simulink model "full_maneuver_platoon"  (R2022a)
settings: Solver=ode23t  StartTime=0.0  StopTime=300  FixedStep=0.1  MaxStep=0.01  RelTol=1e-3
InitFcn:
  | totalVehicles = 7;
  | if exist('vehStatesBus', 'var')==0
  | load vehBuses
  | end
  | if exist('vehErrorsBus', 'var')==0
  | load vehBuses
  | end
libraries: simulink x80, powerlib_meascontrol x16, autolibshared x7, dspsigops x4
(part 2 of 9)

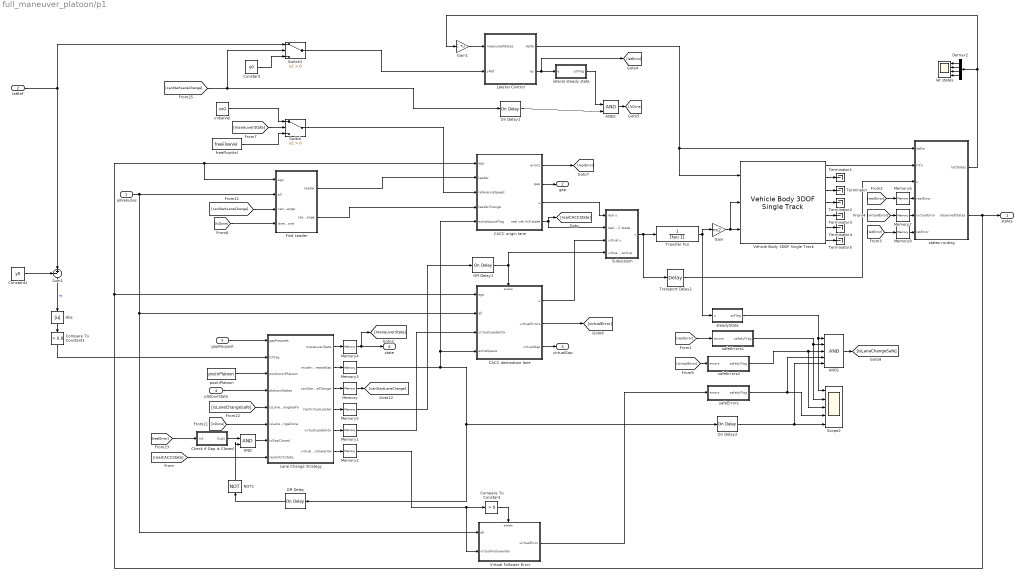
== system full_maneuver_platoon/p1 ==
  allVehicles : Inport
  latRef : Inport  Port=2
  gapRequest : Inport  Port=3
  platoonState : Inport  Port=4
  AND : Logic  IconShape=distinctive  AllPortsSameDT=off  OutDataTypeStr=boolean
  AND1 : Logic  Inputs=5  IconShape=distinctive  AllPortsSameDT=off  OutDataTypeStr=boolean
  AND2 : Logic  IconShape=distinctive  AllPortsSameDT=off  OutDataTypeStr=boolean
  Abs : Abs  SaturateOnIntegerOverflow=off
  CACC destination lane : Subsystem
  CACC origin lane : Subsystem
  Check if Gap is Closed : Subsystem
  Compare To Constant : simulink/Logic and Bit Operations/Compare To Constant  relop=>  const=0  OutDataTypeStr=boolean
  Compare To Constant1 : simulink/Logic and Bit Operations/Compare To Constant  relop=>  const=0.8  OutDataTypeStr=boolean
  Constant : Constant  Value=y0
  Constant1 : Constant  Value=y0
  Demux2 : Demux
  Find Leader : Subsystem
  Gain : Gain  Gain=m/2
  Gain1 : Gain  Gain=C  Multiplication=Matrix(K*u)
  Lane Change Strategy : Subsystem  Variant=on  VariantControlMode=label  LabelModeActiveChoice=leaderFirstInvert
  Lateral Control : Subsystem
  Memory{,1..8} (9 alike) : Memory
  NOT1 : Logic  Operator=NOT  IconShape=distinctive  AllPortsSameDT=off  OutDataTypeStr=boolean
  Off Delay : powerlib_meascontrol/Logic/On Delay  DelayType=Off delay  delay=1  ic=0  Ts=0
  Off Delay1 : powerlib_meascontrol/Logic/On Delay  DelayType=Off delay  delay=1  ic=0  Ts=0
  On Delay1 : powerlib_meascontrol/Logic/On Delay  DelayType=On delay  delay=1  ic=0  Ts=0
  On Delay2 : powerlib_meascontrol/Logic/On Delay  DelayType=On delay  delay=1  ic=0  Ts=0
  Scope2 : Scope  NumInputPorts=5
  Subsystem : Subsystem
  Sum1 : Sum  Inputs=-+|
  Switch : Switch  Criteria=u2 > Threshold  SaturateOnIntegerOverflow=off  InputSameDT=off
  Switch1 : Switch  Criteria=u2 > Threshold  SaturateOnIntegerOverflow=off  InputSameDT=off
  Terminator{,1..5} (6 alike) : Terminator
  Transfer Fcn : TransferFcn  Denominator=[tau 1]
  Transport Delay1 : TransportDelay  DelayTime=0.01
  Vehicle Body 3DOF Single Track : autolibshared/Vehicle Body 3DOF Single Track  trackMode=Single (bicycle)  inputMode=External longitudinal forces  frontSteerMode=on  rearSteerMode=off  windMode=off  muMode=off  extFMode=off  extMMode=off  htchFMode=off  htchMMode=off  extXo=off  extpsio=off  extxdoto=off  extro=off  extYo=off  extTamb=off  extydoto=off  aMode=2  NF=2  NR=2  m=m  a=lf  b=lr  h=0.35  dh=1  hh=0.2  X_o=x0  xdot_o=vx0  CalphaMode=off  sigmaMode=on  d=0  hl=0  w=[1.4,1.4]  Cy_f=12e3  Cy_r=11e3  sigma_f=.1  sigma_r=.1  alpha_f_brk=[-.1 .1]  Cy_f_data=[-9e3 9e3]  alpha_r_brk=[-.1 .1]  Cy_r_data=[-9e3 9e3]  Y_o=y0  ydot_o=0  Izz=4000  psi_o=0  r_o=0  Af=2  Cd=.3  Cl=.1  Cpm=.1  beta_w=[0:0.01:0.3]  Cs=[0:0.03:0.9]  Cym=[0:0.01:0.3]  Pabs=101325  Tair=273  g=9.81  mu=1  xdot_tol=.01  Fznom=5000  Fxtire_sat=7e4  Fytire_sat=7e4  longOff=0  latOff=0  vertOff=0  wrapAng=off
      settings: SourceProductBaseCode=PW,DR,MT,VE
  Virtual Follower Error : Subsystem  TreatAsAtomicUnit=on
  freeFlowVel : Constant  Value=freeFlowVel
  initialVel : Constant  Value=vx0
  lat states : Scope  NumInputPorts=4
  lateral steady state : Subsystem
  posInPlatoon : Constant  Value=posInPlatoon
  safeErrors : Subsystem
  safeErrors1 : Subsystem
  safeErrors2 : Subsystem
  states routing : Subsystem
  steadyState : Subsystem
  states : Outport  VectorParamsAs1DForOutWhenUnconnected=off
  gap : Outport  Port=2  VectorParamsAs1DForOutWhenUnconnected=off
  virtualGap : Outport  Port=3  VectorParamsAs1DForOutWhenUnconnected=off
  state : Outport  Port=4  VectorParamsAs1DForOutWhenUnconnected=off
  wires:
  [realCACCState] -> Lane Change Strategy/8(realCACCstate)
  Memory8/1 -> states routing/6(IatError)
  Memory7/1 -> states routing/5(virtualError)
  Memory6/1 -> states routing/4(realError)
  Memory2/1 -> Virtual Follower Error/2(virtualFollowerIdx), Compare To Constant/1
  gapRequest/1 -> Lane Change Strategy/1(gapRequest)
  Sum1/1 -> Abs/1  "ey"
  Transfer Fcn/1 -> steadyState/1(u), Gain/1
  states routing/2(observedStates) -> states/1, Find Leader/1(ego), CACC origin lane/1(ego), CACC destination lane/1(ego)
  Vehicle Body 3DOF Single Track/3 -> Terminator/1
  Vehicle Body 3DOF Single Track/1 -> states routing/2(Info)
  Gain/1 -> Vehicle Body 3DOF Single Track/3, Vehicle Body 3DOF Single Track/2
  Abs/1 -> Compare To Constant1/1
  allVehicles/1 -> Find Leader/2(all), Virtual Follower Error/1(all), CACC destination lane/2(all)
  platoonState/1 -> Lane Change Strategy/4(platoonStates)
  states routing/1(latStates) -> Gain1/1, Demux2/1
  Gain1/1 -> Lateral Control/1(measuredStates)
  Lateral Control/1(delta) -> Vehicle Body 3DOF Single Track/1, states routing/1(delta)
  Demux2/1 -> lat states/1
  Demux2/2 -> lat states/2
  Demux2/3 -> lat states/3
  Demux2/4 -> lat states/4
  Vehicle Body 3DOF Single Track/2 -> Terminator1/1
  Vehicle Body 3DOF Single Track/4 -> Terminator2/1
  Vehicle Body 3DOF Single Track/5 -> Terminator3/1
  Vehicle Body 3DOF Single Track/6 -> Terminator4/1
  Vehicle Body 3DOF Single Track/7 -> Terminator5/1
  Transport Delay1/1 -> states routing/3(u)
  Compare To Constant1/1 -> Lane Change Strategy/2(lcFlag)
  posInPlatoon/1 -> Lane Change Strategy/3(positionInPlatoon)
  [lcDone] -> Lane Change Strategy/6(isLaneChangeDone)
  [isLaneChangeSafe] -> Lane Change Strategy/5(isLaneChangeSafe)
  [realError] -> Check if Gap is Closed/1(In1)
  Check if Gap is Closed/1(Out1) -> AND/1
  Lane Change Strategy/1(maneuverState) -> Memory4/1
  Lane Change Strategy/2(mustIncreaseGap) -> Memory3/1
  Lane Change Strategy/3(canStartLaneChange) -> Memory/1
  Lane Change Strategy/5(virtualLeaderIdx) -> Memory1/1
  Lane Change Strategy/6(virtualFollowerIdx) -> Memory2/1
  AND/1 -> Lane Change Strategy/7(isGapClosed)
  [canStartLaneChange] -> Find Leader/3(canStartLaneChange)
  [lcDone] -> Find Leader/4(laneChangeDone)
  CACC origin lane/1(errors) -> [realError]
  CACC origin lane/2(gap) -> gap/1
  Memory1/1 -> CACC destination lane/3(virtualLeaderIdx)
  CACC destination lane/2(virtualErrors) -> [virtualError]
  CACC destination lane/3(virtualGap) -> virtualGap/1
  Virtual Follower Error/1(virtualError) -> safeErrors/1(errors)
  [realError] -> safeErrors1/1(errors)
  [virtualError] -> safeErrors2/1(errors)
  safeErrors1/1(safetyFlag) -> Scope2/2, AND1/2
  steadyState/1(ssFlag) -> Scope2/1, AND1/1
  safeErrors2/1(safetyFlag) -> Scope2/3, AND1/3
  AND1/1 -> [isLaneChangeSafe]
  safeErrors/1(safetyFlag) -> Scope2/4, AND1/4
  Memory/1 -> [canStartLaneChange]
  Memory4/1 -> state/1, [maneuverState]
  On Delay2/1 -> Scope2/5, AND1/5
  [maneuverState] -> Switch/2
  freeFlowVel/1 -> Switch/3
  initialVel/1 -> Switch/1
  Switch/1 -> CACC origin lane/3(referenceSpeed)
  NOT1/1 -> AND/2
  Off Delay/1 -> NOT1/1
  Off Delay1/1 -> Subsystem/4(virtual CACC active), CACC destination lane/Enable
  latRef/1 -> Sum1/2, Switch1/1
  Constant/1 -> Switch1/3
  AND2/1 -> [lcDone]
  Lateral Control/2(ey) -> [latError], lateral steady state/1(e)
  [canStartLaneChange] -> Switch1/2, On Delay1/1
  Switch1/1 -> Lateral Control/2(yRef)
  lateral steady state/1(ssFlag) -> AND2/1
  On Delay1/1 -> AND2/2
  Compare To Constant/1 -> Virtual Follower Error/Enable
  Memory5/1 -> Off Delay1/1
  Find Leader/1(leader) -> CACC origin lane/2(leader)
  Find Leader/2(leaderChange) -> CACC origin lane/4(leaderChange)
  Memory3/1 -> On Delay2/1, Off Delay/1, CACC destination lane/4(extraSpace), CACC origin lane/5(extraSpaceFlag)
  Constant1/1 -> Sum1/1
  Lane Change Strategy/4(hasVirtualLeader) -> Memory5/1
  [latError] -> Memory8/1
  [realError] -> Memory6/1
  [virtualError] -> Memory7/1
  CACC origin lane/4(real veh foll state) -> Subsystem/2(real CACC state), [realCACCState]
  Subsystem/1(u) -> Transport Delay1/1, Transfer Fcn/1
  CACC origin lane/3(u) -> Subsystem/1(real u)
  CACC destination lane/1(u) -> Subsystem/3(virtual u)

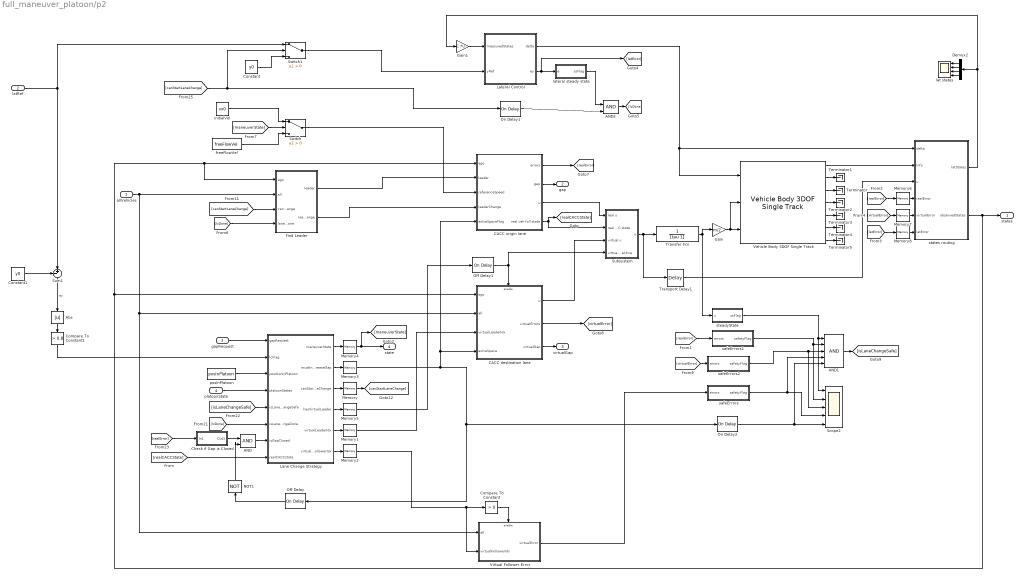
== system full_maneuver_platoon/p2 ==
  allVehicles : Inport
  latRef : Inport  Port=2
  gapRequest : Inport  Port=3
  platoonState : Inport  Port=4
  AND : Logic  IconShape=distinctive  AllPortsSameDT=off  OutDataTypeStr=boolean
  AND1 : Logic  Inputs=5  IconShape=distinctive  AllPortsSameDT=off  OutDataTypeStr=boolean
  AND2 : Logic  IconShape=distinctive  AllPortsSameDT=off  OutDataTypeStr=boolean
  Abs : Abs  SaturateOnIntegerOverflow=off
  CACC destination lane : Subsystem
  CACC origin lane : Subsystem
  Check if Gap is Closed : Subsystem
  Compare To Constant : simulink/Logic and Bit Operations/Compare To Constant  relop=>  const=0  OutDataTypeStr=boolean
  Compare To Constant1 : simulink/Logic and Bit Operations/Compare To Constant  relop=>  const=0.8  OutDataTypeStr=boolean
  Constant : Constant  Value=y0
  Constant1 : Constant  Value=y0
  Demux2 : Demux
  Find Leader : Subsystem
  Gain : Gain  Gain=m/2
  Gain1 : Gain  Gain=C  Multiplication=Matrix(K*u)
  Lane Change Strategy : Subsystem  Variant=on  VariantControlMode=label  LabelModeActiveChoice=leaderFirstInvert
  Lateral Control : Subsystem
  Memory{,1..8} (9 alike) : Memory
  NOT1 : Logic  Operator=NOT  IconShape=distinctive  AllPortsSameDT=off  OutDataTypeStr=boolean
  Off Delay : powerlib_meascontrol/Logic/On Delay  DelayType=Off delay  delay=1  ic=0  Ts=0
  Off Delay1 : powerlib_meascontrol/Logic/On Delay  DelayType=Off delay  delay=1  ic=0  Ts=0
  On Delay1 : powerlib_meascontrol/Logic/On Delay  DelayType=On delay  delay=1  ic=0  Ts=0
  On Delay2 : powerlib_meascontrol/Logic/On Delay  DelayType=On delay  delay=1  ic=0  Ts=0
  Scope2 : Scope  NumInputPorts=5
  Subsystem : Subsystem
  Sum1 : Sum  Inputs=-+|
  Switch : Switch  Criteria=u2 > Threshold  SaturateOnIntegerOverflow=off  InputSameDT=off
  Switch1 : Switch  Criteria=u2 > Threshold  SaturateOnIntegerOverflow=off  InputSameDT=off
  Terminator{,1..5} (6 alike) : Terminator
  Transfer Fcn : TransferFcn  Denominator=[tau 1]
  Transport Delay1 : TransportDelay  DelayTime=0.01
  Vehicle Body 3DOF Single Track : autolibshared/Vehicle Body 3DOF Single Track  trackMode=Single (bicycle)  inputMode=External longitudinal forces  frontSteerMode=on  rearSteerMode=off  windMode=off  muMode=off  extFMode=off  extMMode=off  htchFMode=off  htchMMode=off  extXo=off  extpsio=off  extxdoto=off  extro=off  extYo=off  extTamb=off  extydoto=off  aMode=2  NF=2  NR=2  m=m  a=lf  b=lr  h=0.35  dh=1  hh=0.2  X_o=x0  xdot_o=vx0  CalphaMode=off  sigmaMode=on  d=0  hl=0  w=[1.4,1.4]  Cy_f=12e3  Cy_r=11e3  sigma_f=.1  sigma_r=.1  alpha_f_brk=[-.1 .1]  Cy_f_data=[-9e3 9e3]  alpha_r_brk=[-.1 .1]  Cy_r_data=[-9e3 9e3]  Y_o=y0  ydot_o=0  Izz=4000  psi_o=0  r_o=0  Af=2  Cd=.3  Cl=.1  Cpm=.1  beta_w=[0:0.01:0.3]  Cs=[0:0.03:0.9]  Cym=[0:0.01:0.3]  Pabs=101325  Tair=273  g=9.81  mu=1  xdot_tol=.01  Fznom=5000  Fxtire_sat=7e4  Fytire_sat=7e4  longOff=0  latOff=0  vertOff=0  wrapAng=off
      settings: SourceProductBaseCode=PW,DR,MT,VE
  Virtual Follower Error : Subsystem  TreatAsAtomicUnit=on
  freeFlowVel : Constant  Value=freeFlowVel
  initialVel : Constant  Value=vx0
  lat states : Scope  NumInputPorts=4
  lateral steady state : Subsystem
  posInPlatoon : Constant  Value=posInPlatoon
  safeErrors : Subsystem
  safeErrors1 : Subsystem
  safeErrors2 : Subsystem
  states routing : Subsystem
  steadyState : Subsystem
  states : Outport  VectorParamsAs1DForOutWhenUnconnected=off
  gap : Outport  Port=2  VectorParamsAs1DForOutWhenUnconnected=off
  virtualGap : Outport  Port=3  VectorParamsAs1DForOutWhenUnconnected=off
  state : Outport  Port=4  VectorParamsAs1DForOutWhenUnconnected=off
  wires:
  CACC destination lane/1(u) -> Subsystem/3(virtual u)
  CACC origin lane/3(u) -> Subsystem/1(real u)
  Subsystem/1(u) -> Transfer Fcn/1, Transport Delay1/1
  CACC origin lane/4(real veh foll state) -> [realCACCState], Subsystem/2(real CACC state)
  [virtualError] -> Memory7/1
  [realError] -> Memory6/1
  [latError] -> Memory8/1
  Lane Change Strategy/4(hasVirtualLeader) -> Memory5/1
  Constant1/1 -> Sum1/1
  Memory3/1 -> CACC origin lane/5(extraSpaceFlag), CACC destination lane/4(extraSpace), Off Delay/1, On Delay2/1
  Find Leader/2(leaderChange) -> CACC origin lane/4(leaderChange)
  Find Leader/1(leader) -> CACC origin lane/2(leader)
  Memory5/1 -> Off Delay1/1
  Compare To Constant/1 -> Virtual Follower Error/Enable
  On Delay1/1 -> AND2/2
  lateral steady state/1(ssFlag) -> AND2/1
  Switch1/1 -> Lateral Control/2(yRef)
  [canStartLaneChange] -> On Delay1/1, Switch1/2
  Lateral Control/2(ey) -> lateral steady state/1(e), [latError]
  AND2/1 -> [lcDone]
  Constant/1 -> Switch1/3
  latRef/1 -> Switch1/1, Sum1/2
  Off Delay1/1 -> CACC destination lane/Enable, Subsystem/4(virtual CACC active)
  Off Delay/1 -> NOT1/1
  NOT1/1 -> AND/2
  Switch/1 -> CACC origin lane/3(referenceSpeed)
  initialVel/1 -> Switch/1
  freeFlowVel/1 -> Switch/3
  [maneuverState] -> Switch/2
  On Delay2/1 -> AND1/5, Scope2/5
  Memory4/1 -> [maneuverState], state/1
  Memory/1 -> [canStartLaneChange]
  safeErrors/1(safetyFlag) -> AND1/4, Scope2/4
  AND1/1 -> [isLaneChangeSafe]
  safeErrors2/1(safetyFlag) -> AND1/3, Scope2/3
  steadyState/1(ssFlag) -> AND1/1, Scope2/1
  safeErrors1/1(safetyFlag) -> AND1/2, Scope2/2
  [virtualError] -> safeErrors2/1(errors)
  [realError] -> safeErrors1/1(errors)
  Virtual Follower Error/1(virtualError) -> safeErrors/1(errors)
  CACC destination lane/3(virtualGap) -> virtualGap/1
  CACC destination lane/2(virtualErrors) -> [virtualError]
  Memory1/1 -> CACC destination lane/3(virtualLeaderIdx)
  CACC origin lane/2(gap) -> gap/1
  CACC origin lane/1(errors) -> [realError]
  [lcDone] -> Find Leader/4(laneChangeDone)
  [canStartLaneChange] -> Find Leader/3(canStartLaneChange)
  AND/1 -> Lane Change Strategy/7(isGapClosed)
  Lane Change Strategy/6(virtualFollowerIdx) -> Memory2/1
  Lane Change Strategy/5(virtualLeaderIdx) -> Memory1/1
  Lane Change Strategy/3(canStartLaneChange) -> Memory/1
  Lane Change Strategy/2(mustIncreaseGap) -> Memory3/1
  Lane Change Strategy/1(maneuverState) -> Memory4/1
  Check if Gap is Closed/1(Out1) -> AND/1
  [realError] -> Check if Gap is Closed/1(In1)
  [isLaneChangeSafe] -> Lane Change Strategy/5(isLaneChangeSafe)
  [lcDone] -> Lane Change Strategy/6(isLaneChangeDone)
  posInPlatoon/1 -> Lane Change Strategy/3(positionInPlatoon)
  Compare To Constant1/1 -> Lane Change Strategy/2(lcFlag)
  Transport Delay1/1 -> states routing/3(u)
  Vehicle Body 3DOF Single Track/7 -> Terminator5/1
  Vehicle Body 3DOF Single Track/6 -> Terminator4/1
  Vehicle Body 3DOF Single Track/5 -> Terminator3/1
  Vehicle Body 3DOF Single Track/4 -> Terminator2/1
  Vehicle Body 3DOF Single Track/2 -> Terminator1/1
  Demux2/4 -> lat states/4
  Demux2/3 -> lat states/3
  Demux2/2 -> lat states/2
  Demux2/1 -> lat states/1
  Lateral Control/1(delta) -> states routing/1(delta), Vehicle Body 3DOF Single Track/1
  Gain1/1 -> Lateral Control/1(measuredStates)
  states routing/1(latStates) -> Demux2/1, Gain1/1
  platoonState/1 -> Lane Change Strategy/4(platoonStates)
  allVehicles/1 -> CACC destination lane/2(all), Virtual Follower Error/1(all), Find Leader/2(all)
  Abs/1 -> Compare To Constant1/1
  Gain/1 -> Vehicle Body 3DOF Single Track/2, Vehicle Body 3DOF Single Track/3
  Vehicle Body 3DOF Single Track/1 -> states routing/2(Info)
  Vehicle Body 3DOF Single Track/3 -> Terminator/1
  states routing/2(observedStates) -> CACC destination lane/1(ego), CACC origin lane/1(ego), Find Leader/1(ego), states/1
  Transfer Fcn/1 -> Gain/1, steadyState/1(u)
  Sum1/1 -> Abs/1  "ey"
  gapRequest/1 -> Lane Change Strategy/1(gapRequest)
  Memory2/1 -> Compare To Constant/1, Virtual Follower Error/2(virtualFollowerIdx)
  Memory6/1 -> states routing/4(realError)
  Memory7/1 -> states routing/5(virtualError)
  Memory8/1 -> states routing/6(IatError)
  [realCACCState] -> Lane Change Strategy/8(realCACCstate)

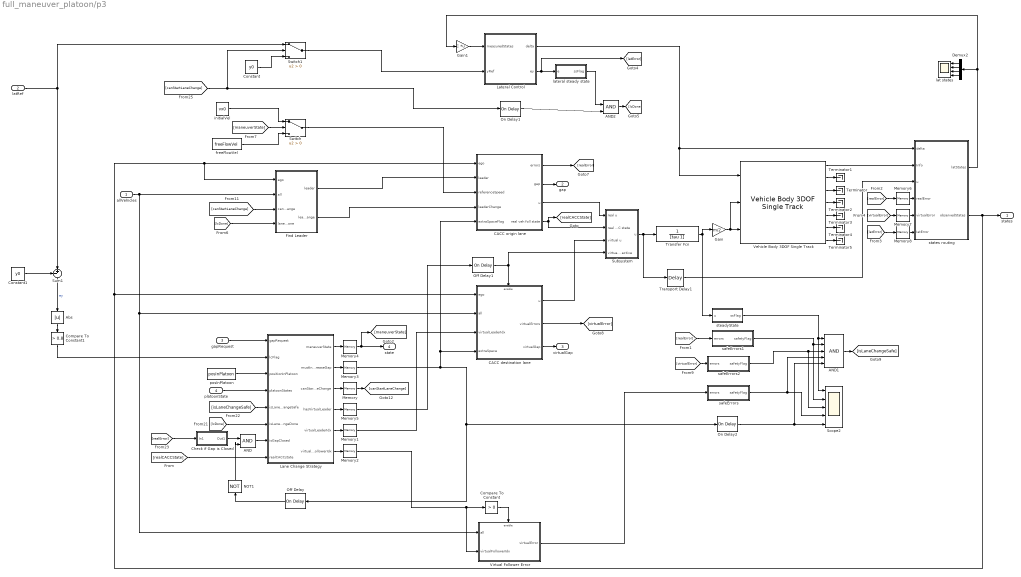
== system full_maneuver_platoon/p3 ==
  allVehicles : Inport
  latRef : Inport  Port=2
  gapRequest : Inport  Port=3
  platoonState : Inport  Port=4
  AND : Logic  IconShape=distinctive  AllPortsSameDT=off  OutDataTypeStr=boolean
  AND1 : Logic  Inputs=5  IconShape=distinctive  AllPortsSameDT=off  OutDataTypeStr=boolean
  AND2 : Logic  IconShape=distinctive  AllPortsSameDT=off  OutDataTypeStr=boolean
  Abs : Abs  SaturateOnIntegerOverflow=off
  CACC destination lane : Subsystem
  CACC origin lane : Subsystem
  Check if Gap is Closed : Subsystem
  Compare To Constant : simulink/Logic and Bit Operations/Compare To Constant  relop=>  const=0  OutDataTypeStr=boolean
  Compare To Constant1 : simulink/Logic and Bit Operations/Compare To Constant  relop=>  const=0.8  OutDataTypeStr=boolean
  Constant : Constant  Value=y0
  Constant1 : Constant  Value=y0
  Demux2 : Demux
  Find Leader : Subsystem
  Gain : Gain  Gain=m/2
  Gain1 : Gain  Gain=C  Multiplication=Matrix(K*u)
  Lane Change Strategy : Subsystem  Variant=on  VariantControlMode=label  LabelModeActiveChoice=leaderFirstInvert
  Lateral Control : Subsystem
  Memory{,1..8} (9 alike) : Memory
  NOT1 : Logic  Operator=NOT  IconShape=distinctive  AllPortsSameDT=off  OutDataTypeStr=boolean
  Off Delay : powerlib_meascontrol/Logic/On Delay  DelayType=Off delay  delay=1  ic=0  Ts=0
  Off Delay1 : powerlib_meascontrol/Logic/On Delay  DelayType=Off delay  delay=1  ic=0  Ts=0
  On Delay1 : powerlib_meascontrol/Logic/On Delay  DelayType=On delay  delay=1  ic=0  Ts=0
  On Delay2 : powerlib_meascontrol/Logic/On Delay  DelayType=On delay  delay=1  ic=0  Ts=0
  Scope2 : Scope  NumInputPorts=5
  Subsystem : Subsystem
  Sum1 : Sum  Inputs=-+|
  Switch : Switch  Criteria=u2 > Threshold  SaturateOnIntegerOverflow=off  InputSameDT=off
  Switch1 : Switch  Criteria=u2 > Threshold  SaturateOnIntegerOverflow=off  InputSameDT=off
  Terminator{,1..5} (6 alike) : Terminator
  Transfer Fcn : TransferFcn  Denominator=[tau 1]
  Transport Delay1 : TransportDelay  DelayTime=0.01
  Vehicle Body 3DOF Single Track : autolibshared/Vehicle Body 3DOF Single Track  trackMode=Single (bicycle)  inputMode=External longitudinal forces  frontSteerMode=on  rearSteerMode=off  windMode=off  muMode=off  extFMode=off  extMMode=off  htchFMode=off  htchMMode=off  extXo=off  extpsio=off  extxdoto=off  extro=off  extYo=off  extTamb=off  extydoto=off  aMode=2  NF=2  NR=2  m=m  a=lf  b=lr  h=0.35  dh=1  hh=0.2  X_o=x0  xdot_o=vx0  CalphaMode=off  sigmaMode=on  d=0  hl=0  w=[1.4,1.4]  Cy_f=12e3  Cy_r=11e3  sigma_f=.1  sigma_r=.1  alpha_f_brk=[-.1 .1]  Cy_f_data=[-9e3 9e3]  alpha_r_brk=[-.1 .1]  Cy_r_data=[-9e3 9e3]  Y_o=y0  ydot_o=0  Izz=4000  psi_o=0  r_o=0  Af=2  Cd=.3  Cl=.1  Cpm=.1  beta_w=[0:0.01:0.3]  Cs=[0:0.03:0.9]  Cym=[0:0.01:0.3]  Pabs=101325  Tair=273  g=9.81  mu=1  xdot_tol=.01  Fznom=5000  Fxtire_sat=7e4  Fytire_sat=7e4  longOff=0  latOff=0  vertOff=0  wrapAng=off
      settings: SourceProductBaseCode=PW,DR,MT,VE
  Virtual Follower Error : Subsystem  TreatAsAtomicUnit=on
  freeFlowVel : Constant  Value=freeFlowVel
  initialVel : Constant  Value=vx0
  lat states : Scope  NumInputPorts=4
  lateral steady state : Subsystem
  posInPlatoon : Constant  Value=posInPlatoon
  safeErrors : Subsystem
  safeErrors1 : Subsystem
  safeErrors2 : Subsystem
  states routing : Subsystem
  steadyState : Subsystem
  states : Outport  VectorParamsAs1DForOutWhenUnconnected=off
  gap : Outport  Port=2  VectorParamsAs1DForOutWhenUnconnected=off
  virtualGap : Outport  Port=3  VectorParamsAs1DForOutWhenUnconnected=off
  state : Outport  Port=4  VectorParamsAs1DForOutWhenUnconnected=off
  wires:
  [realCACCState] -> Lane Change Strategy/8(realCACCstate)
  Memory8/1 -> states routing/6(IatError)
  Memory7/1 -> states routing/5(virtualError)
  Memory6/1 -> states routing/4(realError)
  Memory2/1 -> Virtual Follower Error/2(virtualFollowerIdx), Compare To Constant/1
  gapRequest/1 -> Lane Change Strategy/1(gapRequest)
  Sum1/1 -> Abs/1  "ey"
  Transfer Fcn/1 -> steadyState/1(u), Gain/1
  states routing/2(observedStates) -> states/1, Find Leader/1(ego), CACC origin lane/1(ego), CACC destination lane/1(ego)
  Vehicle Body 3DOF Single Track/3 -> Terminator/1
  Vehicle Body 3DOF Single Track/1 -> states routing/2(Info)
  Gain/1 -> Vehicle Body 3DOF Single Track/3, Vehicle Body 3DOF Single Track/2
  Abs/1 -> Compare To Constant1/1
  allVehicles/1 -> Find Leader/2(all), Virtual Follower Error/1(all), CACC destination lane/2(all)
  platoonState/1 -> Lane Change Strategy/4(platoonStates)
  states routing/1(latStates) -> Gain1/1, Demux2/1
  Gain1/1 -> Lateral Control/1(measuredStates)
  Lateral Control/1(delta) -> Vehicle Body 3DOF Single Track/1, states routing/1(delta)
  Demux2/1 -> lat states/1
  Demux2/2 -> lat states/2
  Demux2/3 -> lat states/3
  Demux2/4 -> lat states/4
  Vehicle Body 3DOF Single Track/2 -> Terminator1/1
  Vehicle Body 3DOF Single Track/4 -> Terminator2/1
  Vehicle Body 3DOF Single Track/5 -> Terminator3/1
  Vehicle Body 3DOF Single Track/6 -> Terminator4/1
  Vehicle Body 3DOF Single Track/7 -> Terminator5/1
  Transport Delay1/1 -> states routing/3(u)
  Compare To Constant1/1 -> Lane Change Strategy/2(lcFlag)
  posInPlatoon/1 -> Lane Change Strategy/3(positionInPlatoon)
  [lcDone] -> Lane Change Strategy/6(isLaneChangeDone)
  [isLaneChangeSafe] -> Lane Change Strategy/5(isLaneChangeSafe)
  [realError] -> Check if Gap is Closed/1(In1)
  Check if Gap is Closed/1(Out1) -> AND/1
  Lane Change Strategy/1(maneuverState) -> Memory4/1
  Lane Change Strategy/2(mustIncreaseGap) -> Memory3/1
  Lane Change Strategy/3(canStartLaneChange) -> Memory/1
  Lane Change Strategy/5(virtualLeaderIdx) -> Memory1/1
  Lane Change Strategy/6(virtualFollowerIdx) -> Memory2/1
  AND/1 -> Lane Change Strategy/7(isGapClosed)
  [canStartLaneChange] -> Find Leader/3(canStartLaneChange)
  [lcDone] -> Find Leader/4(laneChangeDone)
  CACC origin lane/1(errors) -> [realError]
  CACC origin lane/2(gap) -> gap/1
  Memory1/1 -> CACC destination lane/3(virtualLeaderIdx)
  CACC destination lane/2(virtualErrors) -> [virtualError]
  CACC destination lane/3(virtualGap) -> virtualGap/1
  Virtual Follower Error/1(virtualError) -> safeErrors/1(errors)
  [realError] -> safeErrors1/1(errors)
  [virtualError] -> safeErrors2/1(errors)
  safeErrors1/1(safetyFlag) -> Scope2/2, AND1/2
  steadyState/1(ssFlag) -> Scope2/1, AND1/1
  safeErrors2/1(safetyFlag) -> Scope2/3, AND1/3
  AND1/1 -> [isLaneChangeSafe]
  safeErrors/1(safetyFlag) -> Scope2/4, AND1/4
  Memory/1 -> [canStartLaneChange]
  Memory4/1 -> state/1, [maneuverState]
  On Delay2/1 -> Scope2/5, AND1/5
  [maneuverState] -> Switch/2
  freeFlowVel/1 -> Switch/3
  initialVel/1 -> Switch/1
  Switch/1 -> CACC origin lane/3(referenceSpeed)
  NOT1/1 -> AND/2
  Off Delay/1 -> NOT1/1
  Off Delay1/1 -> Subsystem/4(virtual CACC active), CACC destination lane/Enable
  latRef/1 -> Sum1/2, Switch1/1
  Constant/1 -> Switch1/3
  AND2/1 -> [lcDone]
  Lateral Control/2(ey) -> [latError], lateral steady state/1(e)
  [canStartLaneChange] -> Switch1/2, On Delay1/1
  Switch1/1 -> Lateral Control/2(yRef)
  lateral steady state/1(ssFlag) -> AND2/1
  On Delay1/1 -> AND2/2
  Compare To Constant/1 -> Virtual Follower Error/Enable
  Memory5/1 -> Off Delay1/1
  Find Leader/1(leader) -> CACC origin lane/2(leader)
  Find Leader/2(leaderChange) -> CACC origin lane/4(leaderChange)
  Memory3/1 -> On Delay2/1, Off Delay/1, CACC destination lane/4(extraSpace), CACC origin lane/5(extraSpaceFlag)
  Constant1/1 -> Sum1/1
  Lane Change Strategy/4(hasVirtualLeader) -> Memory5/1
  [latError] -> Memory8/1
  [realError] -> Memory6/1
  [virtualError] -> Memory7/1
  CACC origin lane/4(real veh foll state) -> Subsystem/2(real CACC state), [realCACCState]
  Subsystem/1(u) -> Transport Delay1/1, Transfer Fcn/1
  CACC origin lane/3(u) -> Subsystem/1(real u)
  CACC destination lane/1(u) -> Subsystem/3(virtual u)

== system full_maneuver_platoon/Fd/CACC destination lane ==
  ego : Inport
  all : Inport  Port=2
  virtualLeaderIdx : Inport  Port=3
  extraSpace : Inport  Port=4
  Enable : EnablePort
  Demux : Demux  Outputs=2
  Detect Change : simulink/Logic and Bit Operations/Detect Change  vinit=0  OutDataTypeStr=boolean
  Scope virtualLeaderIdx : Scope
  Selector : Selector  InputPortWidth=totalVehicles  IndexOptions=Index vector (port)  Indices=[1]  OutputSizes=1
  Virtual Vehicle Following : Subsystem  TreatAsAtomicUnit=on
  virtual error scope : Scope  NumInputPorts=2
  u : Outport  OutputWhenDisabled=reset  InitialOutput=maxAcceleration+1
  virtualErrors : Outport  Port=2  InitialOutput=[0; 0]
  virtualGap : Outport  Port=3  InitialOutput=[0]
  wires:
  virtualLeaderIdx/1 -> Detect Change/1, Selector/2, Scope virtualLeaderIdx/1
  all/1 -> Selector/1
  Demux/2 -> virtual error scope/2
  Demux/1 -> virtual error scope/1
  ego/1 -> Virtual Vehicle Following/1(ego)
  Virtual Vehicle Following/1(u) -> u/1
  Virtual Vehicle Following/3(virtualGap) -> virtualGap/1
  Virtual Vehicle Following/2(virtualErrors) -> virtualErrors/1, Demux/1
  Detect Change/1 -> Virtual Vehicle Following/3(leaderChange)
  Selector/1 -> Virtual Vehicle Following/2(virtualLeader)
  extraSpace/1 -> Virtual Vehicle Following/4(extraSpaceFlag)

== system full_maneuver_platoon/Fd/CACC origin lane ==
  ego : Inport
  leader : Inport  Port=2
  referenceSpeed : Inport  Port=3
  leaderChange : Inport  Port=4
  extraSpaceFlag : Inport  Port=5
  Controller Real Leader : Subsystem
  Demux : Demux  Outputs=2
  errorScope : Scope  NumInputPorts=2
  errors : Outport
  gap : Outport  Port=2
  u : Outport  Port=3
  wires:
  Demux/2 -> errorScope/2
  Demux/1 -> errorScope/1
  referenceSpeed/1 -> Controller Real Leader/3(referenceSpeed)
  Controller Real Leader/1(u) -> u/1
  ego/1 -> Controller Real Leader/1(ego)
  leader/1 -> Controller Real Leader/2(leader)
  Controller Real Leader/2(errors) -> errors/1, Demux/1
  leaderChange/1 -> Controller Real Leader/4(leaderChange)
  extraSpaceFlag/1 -> Controller Real Leader/5(extraSpaceFlag)
  Controller Real Leader/3(gap) -> gap/1

== system full_maneuver_platoon/Fd/Check if Gap is Closed ==
  In1 : Inport
  AND : Logic  Inputs=1  IconShape=distinctive  AllPortsSameDT=off  OutDataTypeStr=boolean
  Abs2 : Abs  SaturateOnIntegerOverflow=off
  Compare To Constant2 : simulink/Logic and Bit Operations/Compare To Constant  relop=<=  const=1  OutDataTypeStr=boolean
  Mux : Mux  Inputs=2
  Transport Delay2 : TransportDelay
  Out1 : Outport
  wires:
  In1/1 -> Mux/2, Transport Delay2/1
  Mux/1 -> Abs2/1
  Compare To Constant2/1 -> AND/1
  Abs2/1 -> Compare To Constant2/1
  AND/1 -> Out1/1
  Transport Delay2/1 -> Mux/1

== system full_maneuver_platoon/Fd/Find Leader ==
  ego : Inport
  all : Inport  Port=2
  canStartLaneChange : Inport  Port=3
  laneChangeDone : Inport  Port=4
  Detect Change : simulink/Logic and Bit Operations/Detect Change  vinit=0  OutDataTypeStr=boolean
  NOT : Logic  Operator=NOT  IconShape=distinctive  AllPortsSameDT=off  OutDataTypeStr=boolean
  OR : Logic  Operator=OR  IconShape=distinctive  AllPortsSameDT=off  OutDataTypeStr=boolean
  Selector : Selector  InputPortWidth=totalVehicles+1  IndexOptions=Index vector (port)  Indices=[1]  OutputSizes=1
  Subsystem : Subsystem
  Vector Concatenate : Concatenate
  farAwayVeh : Subsystem
  realLeaderIdx : Scope
  leader : Outport  VectorParamsAs1DForOutWhenUnconnected=off
  leaderChange : Outport  Port=2  VectorParamsAs1DForOutWhenUnconnected=off
  wires:
  Detect Change/1 -> leaderChange/1
  Selector/1 -> leader/1
  laneChangeDone/1 -> OR/2
  ego/1 -> Subsystem/1(ego), farAwayVeh/1(ego)
  all/1 -> Vector Concatenate/1, Subsystem/2(all)
  OR/1 -> Subsystem/Enable  "isLaneChanging"
  canStartLaneChange/1 -> NOT/1
  NOT/1 -> OR/1
  Subsystem/1(idx) -> realLeaderIdx/1, Selector/2, Detect Change/1
  farAwayVeh/1(Out1) -> Vector Concatenate/2
  Vector Concatenate/1 -> Selector/1

== system full_maneuver_platoon/Fd/Lane Change Strategy ==
  note: 1) Add Subsystem or Model blocks as valid variant choices.
      | 2) You cannot connect blocks at this level. At simulation, connectivity is automatically
      | determined, based on the active variant and port name matching.
  gapRequest : Inport
  lcFlag : Inport  Port=2
  positionInPlatoon : Inport  Port=3
  platoonStates : Inport  Port=4
  isLaneChangeSafe : Inport  Port=5
  isLaneChangeDone : Inport  Port=6
  isGapClosed : Inport  Port=7
  Strategy 1: synchronous : Subsystem  VariantControl=synchronous
  Strategy 2: leader first : Subsystem  VariantControl=leaderFirst
  Strategy 3: last first : Subsystem  VariantControl=lastFirst
  Strategy 4: leader first invert : Subsystem  VariantControl=leaderFirstInvert
  maneuverState : Outport
  mustIncreaseGap : Outport  Port=2
  canStartLaneChange : Outport  Port=3
  hasVirtualLeader : Outport  Port=4
  virtualLeaderIdx : Outport  Port=5
  virtualFollowerIdx : Outport  Port=6

== system full_maneuver_platoon/Fd/Lateral Control ==
  measuredStates : Inport
  yRef : Inport  Port=2
  Demux2 : Demux
  Full State Observer : Subsystem  Commented=on
  Gain : Gain  Gain=5
  Gain1 : Gain  Gain=Klat  Multiplication=Matrix(K*u)
  Integrator : Integrator  InitialCondition=y0
  Pad : dspsigops/Pad  padAlong=Columns  dimsToPad=1  valSrc=Specify via dialog  padVal=0  spec=Output size  padNumOutRowsSpecMethod=User-specified  numOutRows=4  padNumOutColsSpecMethod=User-specified  numOutCols=1  isVarDimsMode=off  padBeginning=0  padEnd=0  outSizeMode=User-specified  outSize=1  padSigAt=End  trunc_flag=None  roundingMode=Floor  overflowMode=off  truncOrWrapMode=Truncate  wrap_flag=None
      settings: SourceProductBaseCode=DS
  Rate Limiter : RateLimiter  RisingSlewLimit=maxDeltaDot  FallingSlewLimit=-maxDeltaDot  SampleTimeMode=inherited
  Saturation : Saturate  UpperLimit=maxDelta  LowerLimit=-maxDelta
  Saturation1 : Saturate  UpperLimit=2  LowerLimit=-2
  Scope : Scope  NumInputPorts=4
  Scope1 : Scope  NumInputPorts=2
  Selector : Selector  InputPortWidth=4  IndexOptions=Index vector (dialog)  Indices=[1]  OutputSizes=1
  Sum : Sum  Inputs=|+-
  Sum2 : Sum  Inputs=|+-
  delta : Outport  VectorParamsAs1DForOutWhenUnconnected=off
  ey : Outport  Port=2  VectorParamsAs1DForOutWhenUnconnected=off
  wires:
  Rate Limiter/1 -> Full State Observer/2(delta), Scope1/1, delta/1  "delta"
  Demux2/1 -> Scope/1
  Integrator/1 -> Sum2/2, Pad/1
  Gain1/1 -> Scope1/2, Saturation/1
  Sum/1 -> Selector/1, Gain1/1
  Pad/1 -> Sum/1
  Demux2/4 -> Scope/4
  Demux2/2 -> Scope/2
  Sum2/1 -> Gain/1
  Saturation/1 -> Rate Limiter/1
  Demux2/3 -> Scope/3
  yRef/1 -> Sum2/1
  measuredStates/1 -> Full State Observer/1(measuredOutputs), Demux2/1, Sum/2  "estStates"
  Gain/1 -> Saturation1/1
  Saturation1/1 -> Integrator/1
  Selector/1 -> ey/1

== system full_maneuver_platoon/Fd/Virtual Follower Error ==
  ego : Inport
  all : Inport  Port=2
  virtualFollowerIdx : Inport  Port=3
  Enable : EnablePort
  Bus Selector : BusSelector  OutputSignals=X,Xdot
  Bus Selector1 : BusSelector  OutputSignals=X,Xdot
  Multiply : Product
  Mux : Mux  Inputs=2
  Scope : Scope
  Selector1 : Selector  InputPortWidth=totalVehicles  IndexOptions=Index vector (port)  Indices=[1]  OutputSizes=1
  Sum : Sum  Inputs=-+|
  Sum1 : Sum  Inputs=++|
  Sum2 : Sum  Inputs=+-|
  Sum3 : Sum  Inputs=|++
  Sum4 : Sum  Inputs=-+|
  d0 : Constant  Value=d0
  h : Constant  Value=h
  vLen : Constant  Value=lr+lf
  virtual follower scope : Scope  NumInputPorts=2
  virtualError : Outport  InitialOutput=[0; 0]
  wires:
  Sum4/1 -> Mux/2, virtual follower scope/2
  Bus Selector/2 -> Sum4/1, Multiply/1  "<Xdot>"
  Sum3/1 -> Sum2/2  "desired  gap"
  ego/1 -> Bus Selector1/1
  Sum1/1 -> Sum/1  "x (front bumber)"
  Sum/1 -> Sum2/1  "gap"
  vLen/1 -> Sum1/1
  Bus Selector/1 -> Sum1/2  "<X>"
  Bus Selector1/1 -> Sum/2  "<X>"
  Multiply/1 -> Sum3/1
  Sum2/1 -> Mux/1, virtual follower scope/1
  Selector1/1 -> Bus Selector/1
  Bus Selector1/2 -> Sum4/2  "<Xdot>"
  h/1 -> Multiply/2  "time headway"
  d0/1 -> Sum3/2  "gap at  standstill"
  Mux/1 -> virtualError/1
  virtualFollowerIdx/1 -> Selector1/2, Scope/1
  all/1 -> Selector1/1

== system full_maneuver_platoon/Fd/lateral steady state ==
  e : Inport
  AND : Logic  IconShape=distinctive  AllPortsSameDT=off  OutDataTypeStr=boolean
  Abs2 : Abs  SaturateOnIntegerOverflow=off
  Compare To Constant2 : simulink/Logic and Bit Operations/Compare To Constant  relop=<=  const=0.1  OutDataTypeStr=boolean
  Demux : Demux  Outputs=2
  Mux : Mux  Inputs=2
  Transport Delay2 : TransportDelay
  ssFlag : Outport  VectorParamsAs1DForOutWhenUnconnected=off
  wires:
  e/1 -> Transport Delay2/1, Mux/2
  Abs2/1 -> Compare To Constant2/1
  Demux/1 -> AND/1
  Transport Delay2/1 -> Mux/1
  AND/1 -> ssFlag/1
  Compare To Constant2/1 -> Demux/1
  Mux/1 -> Abs2/1
  Demux/2 -> AND/2

== system full_maneuver_platoon/Fd/safeErrors ==
  errors : Inport
  AND : Logic  Inputs=1  IconShape=distinctive  AllPortsSameDT=off  OutDataTypeStr=boolean
  Compare To Constant4 : simulink/Logic and Bit Operations/Compare To Constant  relop=>=  const=-0.1  OutDataTypeStr=boolean
  safetyFlag : Outport  VectorParamsAs1DForOutWhenUnconnected=off
  wires:
  AND/1 -> safetyFlag/1
  errors/1 -> Compare To Constant4/1
  Compare To Constant4/1 -> AND/1

== system full_maneuver_platoon/Fd/safeErrors1 ==
  errors : Inport
  AND : Logic  Inputs=1  IconShape=distinctive  AllPortsSameDT=off  OutDataTypeStr=boolean
  Compare To Constant4 : simulink/Logic and Bit Operations/Compare To Constant  relop=>=  const=-0.3  OutDataTypeStr=boolean
  safetyFlag : Outport  VectorParamsAs1DForOutWhenUnconnected=off
  wires:
  AND/1 -> safetyFlag/1
  errors/1 -> Compare To Constant4/1
  Compare To Constant4/1 -> AND/1

== system full_maneuver_platoon/Fd/safeErrors2 ==
  errors : Inport
  AND : Logic  Inputs=1  IconShape=distinctive  AllPortsSameDT=off  OutDataTypeStr=boolean
  Compare To Constant4 : simulink/Logic and Bit Operations/Compare To Constant  relop=>=  const=-0.3  OutDataTypeStr=boolean
  safetyFlag : Outport  VectorParamsAs1DForOutWhenUnconnected=off
  wires:
  errors/1 -> Compare To Constant4/1
  AND/1 -> safetyFlag/1
  Compare To Constant4/1 -> AND/1

== system full_maneuver_platoon/Fd/states routing ==
  delta : Inport
  Info : Inport  Port=2
  u : Inport  Port=3
  realError : Inport  Port=4
  virtualError : Inport  Port=5
  IatError : Inport  Port=6
  Bus Creator : BusCreator  Inputs=12  OutDataTypeStr=Bus: vehStatesBus  NonVirtualBus=on
      settings: InheritFromInputs=off
  Bus Selector : BusSelector  OutputSignals=BdyFrm.Cg.Vel.ydot,BdyFrm.Cg.AngVel.r,InertFrm.RearAxl.Disp.X,InertFrm.Cg.Disp.Y,InertFrm.RearAxl.Vel.Xdot,BdyFrm.Cg.Acc.xddot,InertFrm.Cg.Ang.psi
  Demux : Demux  Outputs=2
  Demux1 : Demux  Outputs=2
  Mux : Mux
  latStates : Outport
  observedStates : Outport  Port=2
  wires:
  IatError/1 -> Bus Creator/12
  Demux1/2 -> Bus Creator/11
  Demux1/1 -> Bus Creator/10
  Demux/2 -> Bus Creator/9
  Demux/1 -> Bus Creator/8
  virtualError/1 -> Demux1/1
  realError/1 -> Demux/1
  Bus Creator/1 -> observedStates/1
  Bus Selector/2 -> Mux/4  "<r>"
  Bus Selector/1 -> Mux/2  "<ydot>"
  Mux/1 -> latStates/1
  delta/1 -> Bus Creator/7
  u/1 -> Bus Creator/6
  Bus Selector/7 -> Bus Creator/5, Mux/3  "<psi>"
  Bus Selector/6 -> Bus Creator/4  "<xddot>"
  Bus Selector/5 -> Bus Creator/3  "<Xdot>"
  Bus Selector/4 -> Mux/1, Bus Creator/2  "<Y>"
  Bus Selector/3 -> Bus Creator/1  "<X>"
  Info/1 -> Bus Selector/1

== system full_maneuver_platoon/Fd/steadyState ==
  u : Inport
  AND : Logic  Inputs=1  IconShape=distinctive  AllPortsSameDT=off  OutDataTypeStr=boolean
  Abs2 : Abs  SaturateOnIntegerOverflow=off
  Compare To Constant2 : simulink/Logic and Bit Operations/Compare To Constant  relop=<=  const=0.2  OutDataTypeStr=boolean
  Mux : Mux  Inputs=2
  Transport Delay2 : TransportDelay
  ssFlag : Outport  VectorParamsAs1DForOutWhenUnconnected=off
  wires:
  Mux/1 -> Abs2/1
  AND/1 -> ssFlag/1
  Transport Delay2/1 -> Mux/1
  Abs2/1 -> Compare To Constant2/1
  u/1 -> Mux/2, Transport Delay2/1
  Compare To Constant2/1 -> AND/1

== system full_maneuver_platoon/Fo/CACC origin lane ==
  ego : Inport
  leader : Inport  Port=2
  referenceSpeed : Inport  Port=3
  leaderChange : Inport  Port=4
  extraSpaceFlag : Inport  Port=5
  Controller Real Leader : Subsystem
  Demux : Demux  Outputs=2
  errorScope : Scope  NumInputPorts=2
  errors : Outport
  gap : Outport  Port=2
  u : Outport  Port=3
  wires:
  Controller Real Leader/3(gap) -> gap/1
  extraSpaceFlag/1 -> Controller Real Leader/5(extraSpaceFlag)
  leaderChange/1 -> Controller Real Leader/4(leaderChange)
  Controller Real Leader/2(errors) -> Demux/1, errors/1
  leader/1 -> Controller Real Leader/2(leader)
  ego/1 -> Controller Real Leader/1(ego)
  Controller Real Leader/1(u) -> u/1
  referenceSpeed/1 -> Controller Real Leader/3(referenceSpeed)
  Demux/1 -> errorScope/1
  Demux/2 -> errorScope/2

== system full_maneuver_platoon/Fo/findLeader ==
  ego : Inport
  all : Inport  Port=2
  lcFlag : Inport  Port=3
  state : Inport  Port=4
  Compare To Constant : simulink/Logic and Bit Operations/Compare To Constant  relop=~=  const=4  OutDataTypeStr=boolean
  Detect Change : simulink/Logic and Bit Operations/Detect Change  vinit=0  OutDataTypeStr=boolean
  NOT : Logic  Operator=NOT  IconShape=distinctive  AllPortsSameDT=off  OutDataTypeStr=boolean
  OR : Logic  Operator=OR  IconShape=distinctive  AllPortsSameDT=off  OutDataTypeStr=boolean
  Selector : Selector  InputPortWidth=totalVehicles+1  IndexOptions=Index vector (port)  Indices=[1]  OutputSizes=1
  Subsystem : Subsystem
  Vector Concatenate : Concatenate
  farAwayVeh : Subsystem
  realLeaderIdx : Scope
  leader : Outport  VectorParamsAs1DForOutWhenUnconnected=off
  leaderChange : Outport  Port=2  InitialOutput=1  VectorParamsAs1DForOutWhenUnconnected=off
  wires:
  Compare To Constant/1 -> OR/2
  state/1 -> Compare To Constant/1
  ego/1 -> Subsystem/1(ego), farAwayVeh/1(ego)
  all/1 -> Subsystem/2(all), Vector Concatenate/1
  Subsystem/1(idx) -> realLeaderIdx/1, Selector/2, Detect Change/1
  OR/1 -> Subsystem/Enable
  lcFlag/1 -> NOT/1
  NOT/1 -> OR/1
  Selector/1 -> leader/1
  farAwayVeh/1(Out1) -> Vector Concatenate/2
  Vector Concatenate/1 -> Selector/1
  Detect Change/1 -> leaderChange/1

== system full_maneuver_platoon/Fo/states routing1 ==
  delta : Inport
  Info : Inport  Port=2
  u : Inport  Port=3
  realError : Inport  Port=4
  virtualError : Inport  Port=5
  IatError : Inport  Port=6
  Bus Creator : BusCreator  Inputs=12  OutDataTypeStr=Bus: vehStatesBus  NonVirtualBus=on
      settings: InheritFromInputs=off
  Bus Selector : BusSelector  OutputSignals=BdyFrm.Cg.Vel.ydot,BdyFrm.Cg.AngVel.r,InertFrm.RearAxl.Disp.X,InertFrm.Cg.Disp.Y,InertFrm.RearAxl.Vel.Xdot,BdyFrm.Cg.Acc.xddot,InertFrm.Cg.Ang.psi
  Demux : Demux  Outputs=2
  Demux1 : Demux  Outputs=2
  Mux : Mux
  latStates : Outport
  observedStates : Outport  Port=2
  wires:
  IatError/1 -> Bus Creator/12
  Demux1/2 -> Bus Creator/11
  Demux1/1 -> Bus Creator/10
  Demux/2 -> Bus Creator/9
  Demux/1 -> Bus Creator/8
  virtualError/1 -> Demux1/1
  realError/1 -> Demux/1
  Bus Creator/1 -> observedStates/1
  Bus Selector/2 -> Mux/4  "<r>"
  Bus Selector/1 -> Mux/2  "<ydot>"
  Mux/1 -> latStates/1
  delta/1 -> Bus Creator/7
  u/1 -> Bus Creator/6
  Bus Selector/7 -> Bus Creator/5, Mux/3  "<psi>"
  Bus Selector/6 -> Bus Creator/4  "<xddot>"
  Bus Selector/5 -> Bus Creator/3  "<Xdot>"
  Bus Selector/4 -> Mux/1, Bus Creator/2  "<Y>"
  Bus Selector/3 -> Bus Creator/1  "<X>"
  Info/1 -> Bus Selector/1

== system full_maneuver_platoon/Ld/CACC origin lane ==
  ego : Inport
  leader : Inport  Port=2
  referenceSpeed : Inport  Port=3
  leaderChange : Inport  Port=4
  extraSpaceFlag : Inport  Port=5
  Controller Real Leader : Subsystem
  Demux : Demux  Outputs=2
  errorScope : Scope  NumInputPorts=2
  errors : Outport
  gap : Outport  Port=2
  u : Outport  Port=3
  wires:
  Controller Real Leader/3(gap) -> gap/1
  extraSpaceFlag/1 -> Controller Real Leader/5(extraSpaceFlag)
  leaderChange/1 -> Controller Real Leader/4(leaderChange)
  Controller Real Leader/2(errors) -> Demux/1, errors/1
  leader/1 -> Controller Real Leader/2(leader)
  ego/1 -> Controller Real Leader/1(ego)
  Controller Real Leader/1(u) -> u/1
  referenceSpeed/1 -> Controller Real Leader/3(referenceSpeed)
  Demux/1 -> errorScope/1
  Demux/2 -> errorScope/2

== system full_maneuver_platoon/Ld/findLeader ==
  ego : Inport
  all : Inport  Port=2
  lcFlag : Inport  Port=3
  state : Inport  Port=4
  Compare To Constant : simulink/Logic and Bit Operations/Compare To Constant  relop=~=  const=4  OutDataTypeStr=boolean
  Detect Change : simulink/Logic and Bit Operations/Detect Change  vinit=0  OutDataTypeStr=boolean
  NOT : Logic  Operator=NOT  IconShape=distinctive  AllPortsSameDT=off  OutDataTypeStr=boolean
  OR : Logic  Operator=OR  IconShape=distinctive  AllPortsSameDT=off  OutDataTypeStr=boolean
  Selector : Selector  InputPortWidth=totalVehicles+1  IndexOptions=Index vector (port)  Indices=[1]  OutputSizes=1
  Subsystem : Subsystem
  Vector Concatenate : Concatenate
  farAwayVeh : Subsystem
  realLeaderIdx : Scope
  leader : Outport  VectorParamsAs1DForOutWhenUnconnected=off
  leaderChange : Outport  Port=2  InitialOutput=1  VectorParamsAs1DForOutWhenUnconnected=off
  wires:
  Compare To Constant/1 -> OR/2
  state/1 -> Compare To Constant/1
  ego/1 -> Subsystem/1(ego), farAwayVeh/1(ego)
  all/1 -> Subsystem/2(all), Vector Concatenate/1
  Subsystem/1(idx) -> realLeaderIdx/1, Selector/2, Detect Change/1
  OR/1 -> Subsystem/Enable
  lcFlag/1 -> NOT/1
  NOT/1 -> OR/1
  Selector/1 -> leader/1
  farAwayVeh/1(Out1) -> Vector Concatenate/2
  Vector Concatenate/1 -> Selector/1
  Detect Change/1 -> leaderChange/1

== system full_maneuver_platoon/Ld/states routing1 ==
  delta : Inport
  Info : Inport  Port=2
  u : Inport  Port=3
  realError : Inport  Port=4
  virtualError : Inport  Port=5
  IatError : Inport  Port=6
  Bus Creator : BusCreator  Inputs=12  OutDataTypeStr=Bus: vehStatesBus  NonVirtualBus=on
      settings: InheritFromInputs=off
  Bus Selector : BusSelector  OutputSignals=BdyFrm.Cg.Vel.ydot,BdyFrm.Cg.AngVel.r,InertFrm.RearAxl.Disp.X,InertFrm.Cg.Disp.Y,InertFrm.RearAxl.Vel.Xdot,BdyFrm.Cg.Acc.xddot,InertFrm.Cg.Ang.psi
  Demux : Demux  Outputs=2
  Demux1 : Demux  Outputs=2
  Mux : Mux
  latStates : Outport
  observedStates : Outport  Port=2
  wires:
  IatError/1 -> Bus Creator/12
  Demux1/2 -> Bus Creator/11
  Demux1/1 -> Bus Creator/10
  Demux/2 -> Bus Creator/9
  Demux/1 -> Bus Creator/8
  virtualError/1 -> Demux1/1
  realError/1 -> Demux/1
  Bus Creator/1 -> observedStates/1
  Bus Selector/2 -> Mux/4  "<r>"
  Bus Selector/1 -> Mux/2  "<ydot>"
  Mux/1 -> latStates/1
  delta/1 -> Bus Creator/7
  u/1 -> Bus Creator/6
  Bus Selector/7 -> Bus Creator/5, Mux/3  "<psi>"
  Bus Selector/6 -> Bus Creator/4  "<xddot>"
  Bus Selector/5 -> Bus Creator/3  "<Xdot>"
  Bus Selector/4 -> Mux/1, Bus Creator/2  "<Y>"
  Bus Selector/3 -> Bus Creator/1  "<X>"
  Info/1 -> Bus Selector/1

== system full_maneuver_platoon/Lo/CACC origin lane ==
  ego : Inport
  leader : Inport  Port=2
  referenceSpeed : Inport  Port=3
  leaderChange : Inport  Port=4
  extraSpaceFlag : Inport  Port=5
  Controller Real Leader : Subsystem
  Demux : Demux  Outputs=2
  errorScope : Scope  NumInputPorts=2
  errors : Outport
  gap : Outport  Port=2
  u : Outport  Port=3
  wires:
  Demux/2 -> errorScope/2
  Demux/1 -> errorScope/1
  referenceSpeed/1 -> Controller Real Leader/3(referenceSpeed)
  Controller Real Leader/1(u) -> u/1
  ego/1 -> Controller Real Leader/1(ego)
  leader/1 -> Controller Real Leader/2(leader)
  Controller Real Leader/2(errors) -> errors/1, Demux/1
  leaderChange/1 -> Controller Real Leader/4(leaderChange)
  extraSpaceFlag/1 -> Controller Real Leader/5(extraSpaceFlag)
  Controller Real Leader/3(gap) -> gap/1

== system full_maneuver_platoon/Lo/findLeader ==
  ego : Inport
  all : Inport  Port=2
  lcFlag : Inport  Port=3
  state : Inport  Port=4
  Compare To Constant : simulink/Logic and Bit Operations/Compare To Constant  relop=~=  const=4  OutDataTypeStr=boolean
  Detect Change : simulink/Logic and Bit Operations/Detect Change  vinit=0  OutDataTypeStr=boolean
  NOT : Logic  Operator=NOT  IconShape=distinctive  AllPortsSameDT=off  OutDataTypeStr=boolean
  OR : Logic  Operator=OR  IconShape=distinctive  AllPortsSameDT=off  OutDataTypeStr=boolean
  Selector : Selector  InputPortWidth=totalVehicles+1  IndexOptions=Index vector (port)  Indices=[1]  OutputSizes=1
  Subsystem : Subsystem
  Vector Concatenate : Concatenate
  farAwayVeh : Subsystem
  realLeaderIdx : Scope
  leader : Outport  VectorParamsAs1DForOutWhenUnconnected=off
  leaderChange : Outport  Port=2  InitialOutput=1  VectorParamsAs1DForOutWhenUnconnected=off
  wires:
  Detect Change/1 -> leaderChange/1
  Vector Concatenate/1 -> Selector/1
  farAwayVeh/1(Out1) -> Vector Concatenate/2
  Selector/1 -> leader/1
  NOT/1 -> OR/1
  lcFlag/1 -> NOT/1
  OR/1 -> Subsystem/Enable
  Subsystem/1(idx) -> Detect Change/1, Selector/2, realLeaderIdx/1
  all/1 -> Vector Concatenate/1, Subsystem/2(all)
  ego/1 -> farAwayVeh/1(ego), Subsystem/1(ego)
  state/1 -> Compare To Constant/1
  Compare To Constant/1 -> OR/2

== system full_maneuver_platoon/Lo/states routing1 ==
  delta : Inport
  Info : Inport  Port=2
  u : Inport  Port=3
  realError : Inport  Port=4
  virtualError : Inport  Port=5
  IatError : Inport  Port=6
  Bus Creator : BusCreator  Inputs=12  OutDataTypeStr=Bus: vehStatesBus  NonVirtualBus=on
      settings: InheritFromInputs=off
  Bus Selector : BusSelector  OutputSignals=BdyFrm.Cg.Vel.ydot,BdyFrm.Cg.AngVel.r,InertFrm.RearAxl.Disp.X,InertFrm.Cg.Disp.Y,InertFrm.RearAxl.Vel.Xdot,BdyFrm.Cg.Acc.xddot,InertFrm.Cg.Ang.psi
  Demux : Demux  Outputs=2
  Demux1 : Demux  Outputs=2
  Mux : Mux
  latStates : Outport
  observedStates : Outport  Port=2
  wires:
  Info/1 -> Bus Selector/1
  Bus Selector/3 -> Bus Creator/1  "<X>"
  Bus Selector/4 -> Bus Creator/2, Mux/1  "<Y>"
  Bus Selector/5 -> Bus Creator/3  "<Xdot>"
  Bus Selector/6 -> Bus Creator/4  "<xddot>"
  Bus Selector/7 -> Mux/3, Bus Creator/5  "<psi>"
  u/1 -> Bus Creator/6
  delta/1 -> Bus Creator/7
  Mux/1 -> latStates/1
  Bus Selector/1 -> Mux/2  "<ydot>"
  Bus Selector/2 -> Mux/4  "<r>"
  Bus Creator/1 -> observedStates/1
  realError/1 -> Demux/1
  virtualError/1 -> Demux1/1
  Demux/1 -> Bus Creator/8
  Demux/2 -> Bus Creator/9
  Demux1/1 -> Bus Creator/10
  Demux1/2 -> Bus Creator/11
  IatError/1 -> Bus Creator/12

== system full_maneuver_platoon/p1/CACC destination lane ==
  ego : Inport
  all : Inport  Port=2
  virtualLeaderIdx : Inport  Port=3
  extraSpace : Inport  Port=4
  Enable : EnablePort
  Demux : Demux  Outputs=2
  Detect Change : simulink/Logic and Bit Operations/Detect Change  vinit=0  OutDataTypeStr=boolean
  Scope virtualLeaderIdx : Scope
  Selector : Selector  InputPortWidth=totalVehicles  IndexOptions=Index vector (port)  Indices=[1]  OutputSizes=1
  Subsystem : Subsystem  Commented=through
  Virtual Vehicle Following : Subsystem  TreatAsAtomicUnit=on
  virtual error scope : Scope  NumInputPorts=2
  u : Outport  OutputWhenDisabled=reset  InitialOutput=maxAcceleration+1
  virtualErrors : Outport  Port=2  InitialOutput=[0; 0]
  virtualGap : Outport  Port=3  InitialOutput=[0]
  wires:
  extraSpace/1 -> Virtual Vehicle Following/4(extraSpaceFlag)
  Selector/1 -> Virtual Vehicle Following/2(virtualLeader)
  Detect Change/1 -> Virtual Vehicle Following/3(leaderChange)
  Virtual Vehicle Following/2(virtualErrors) -> Demux/1, virtualErrors/1
  Virtual Vehicle Following/3(virtualGap) -> virtualGap/1
  Virtual Vehicle Following/1(u) -> Subsystem/1(u)
  ego/1 -> Virtual Vehicle Following/1(ego)
  Demux/1 -> virtual error scope/1
  Demux/2 -> virtual error scope/2
  all/1 -> Selector/1
  virtualLeaderIdx/1 -> Scope virtualLeaderIdx/1, Selector/2, Detect Change/1
  Subsystem/1(u smooth) -> u/1
